simulink model "Switch"  (R2024b)
settings: Solver=VariableStepAuto  StartTime=0.0  StopTime=1  FixedStep=50e-6  MaxStep=0.001  MinStep=1e-8
model workspace (MAT data in the model file):
  condition : Simulink.Parameter (value not decoded)
undefined symbols (not defined in the file or in its folder): DiscIntNeverNeededParam, ee_sli_rtmsupport, gcbh
libraries: spsIdealSwitchLib x12, spsCurrentMeasurementLib x6, spsSeriesRLCBranchLib x6, eeGeneralControl x6, spsControlledVoltageSourceLib x6, spsVoltageMeasurementLib x6, simulink x3, spsAsynchronousMachineSIUnitsLib x2, spsGroundLib x2, spsThreePhaseTransformerInductanceMatrixTypeTwoWindingsLib x1, spspowerguiLib x1
(part 2 of 2)

== matlab function Switch/MATLAB Function ==
  data: output1 output; output2 output; condition input; output3 output; output4 output
function [output1, output2, output3, output4] = multiOutputSwitch(condition)
    
    % Initialize the outputs to specific values (e.g., 0 or NaN) for Simulink to infer size
    output1 = NaN;  % ✅ Fixed: NaN (uppercase N)
    output2 = NaN;  % ✅ Fixed: NaN (uppercase N)
    output3 = NaN;  % ✅ Fixed: NaN (uppercase N)
    output4 = NaN;  % ✅ Fixed: NaN (uppercase N)

    % Check the condition and assign outputs
    switch condition
        case 1
            output1 = 1;
        case 2
            output2 = 1;
        case 3
            output1 = 1;
            output2 = 1;
        case 4
            output3 = 1;
        case 5
            output4 = 1;
        case 6
            output3 = 1;  
            output4 = 1;
        case 7
            output1 = 1;  
            output3 = 1;
        case 8
            output1 = 1;  
            output4 = 1;
        case 9
            output3 = 1;  
            output2 = 1;
        case 10
            output2 = 1;  
            output4 = 1;
        case 11
            output3 = 1;  
            output4 = 1;
            output1 = 1;
        case 12
            output2 = 1;  
            output4 = 1;
            output1 = 1;
        case 13
            output3 = 1;  
            output2 = 1;
            output1 = 1;
        case 14
            output2 = 1;  
            output4 = 1;
            output3 = 1;
        case 15
            output3 = 1;  
            output4 = 1;
            output2 = 1;
            output1 = 1;
        otherwise
            % Handle other conditions or keep the default (NaN) initialization
            output1 = NaN;
            output2 = NaN;
            output3 = NaN;
            output4 = NaN;
    end
end
